simulink model "PrinterMotorPMatlab"  (R2015b)
settings: Solver=FixedStepAuto  StartTime=0.0  StopTime=50  FixedStep=paso  RelTol=1e-3
values from neighbouring files (symbols this model uses):
  MaxAmp = 10    [GeneticPrinterMotor.m]    (also in GeneticPrinterMotor_2_Redefinition.m; GeneticPrinterMotor_3_SelectionCrossoverAdjust.m; GeneticPrinterMotor_4_MicroGA.m; GeneticSnakeP.m)
settings Model: Creator=Christian Dos Santos  LastModifiedBy=Christian Dos Santos

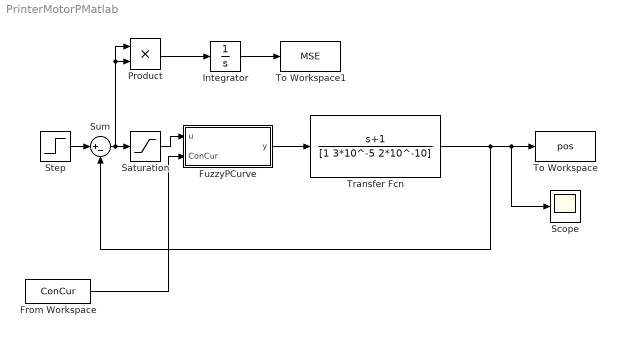
== system PrinterMotorPMatlab ==
  From Workspace : FromWorkspace  VariableName=ConCur  SampleTime=0
  FuzzyPCurve : MATLAB Function  TreatAsAtomicUnit=on
  Integrator : Integrator
  Product : Product
  Saturation : Saturate  UpperLimit=19.99  LowerLimit=-20
  Scope : Scope
  Step : Step  After=MaxAmp  SampleTime=0
  Sum : Sum  Inputs=|+-
  To Workspace : ToWorkspace  VariableName=pos  SampleTime=-1
  To Workspace1 : ToWorkspace  VariableName=MSE  SampleTime=-1
  Transfer Fcn : TransferFcn  Numerator=[1 1]  Denominator=[1 3*10^-5 2*10^-10]
  wires:
  FuzzyPCurve/1(y) -> Transfer Fcn/1
  Step/1 -> Sum/1
  Transfer Fcn/1 -> Scope/1, To Workspace/1, Sum/2
  From Workspace/1 -> FuzzyPCurve/2(ConCur)
  Saturation/1 -> FuzzyPCurve/1(u)
  Sum/1 -> Product/1, Product/2, Saturation/1
  Integrator/1 -> To Workspace1/1
  Product/1 -> Integrator/1

== matlab function PrinterMotorPMatlab/FuzzyPCurve ==
  data: u input; y output; ConCur input
function y = fcn(u, ConCur)
%#codegen
paso = 0.01;
uAux = floor( (u + 20)/ paso + 1 );
y = ConCur(uAux);
